simulink model "Q2"  (R2018a)
settings: Solver=VariableStepAuto  StartTime=0.0  StopTime=10  RelTol=1e-3
libraries: simulink x1
settings Model: Creator=Rodrigo  LastModifiedBy=Rodrigo

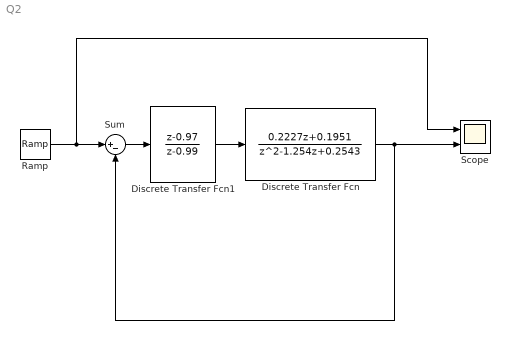
== system Q2 ==
  Discrete Transfer Fcn : DiscreteTransferFcn  Numerator=[0.2227 0.1951]  Denominator=[1 -1.254 0.2543]  SampleTime=0.2
  Discrete Transfer Fcn1 : DiscreteTransferFcn  Numerator=[1 -0.97]  Denominator=[1 -0.99]
  Ramp : simulink/Sources/Ramp  slope=1  start=0  InitialOutput=0
  Scope : Scope  NumInputPorts=2
  Sum : Sum  Inputs=|+-
  wires:
  Discrete Transfer Fcn/1 -> Sum/2, Scope/2
  Ramp/1 -> Scope/1, Sum/1
  Sum/1 -> Discrete Transfer Fcn1/1
  Discrete Transfer Fcn1/1 -> Discrete Transfer Fcn/1
